simulink model "regulacion_nominal_modelo_no_lineal"  (R2021a)
settings: Solver=VariableStepAuto  StartTime=0.0  StopTime=15  RelTol=1e-3
settings Model: Creator=jmata  LastModifiedBy=jmata

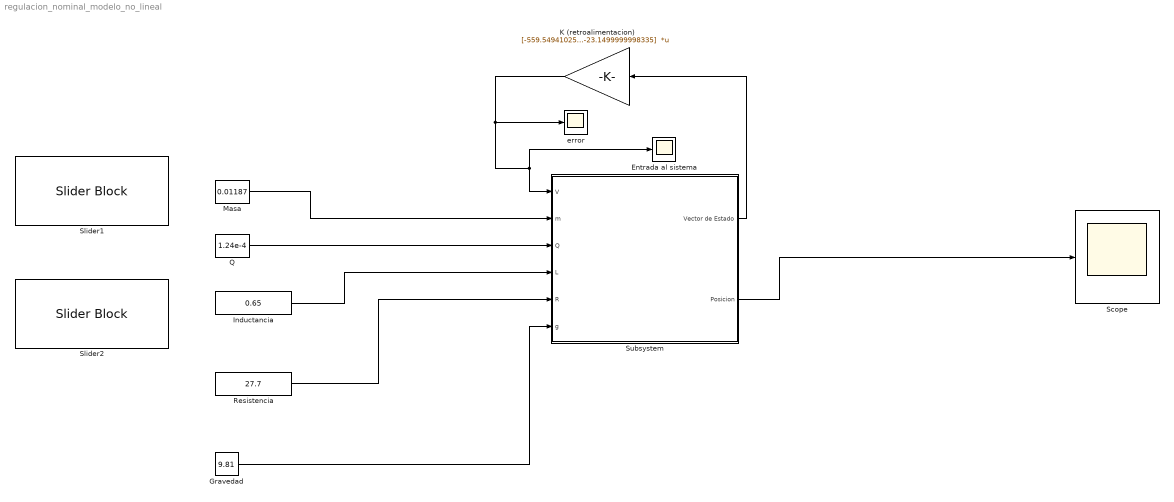
== system regulacion_nominal_modelo_no_lineal ==
  Entrada al sistema : Scope
  Gravedad : Constant  Value=9.81
  Inductancia : Constant  Value=0.65
  K (retroalimentacion) : Gain  Gain=[-559.549410259276, -81.2758440000597, -23.1499999998335]  Multiplication=Matrix(K*u)
  Masa : Constant  Value=0.01187
  Q : Constant  Value=1.24e-4
  Resistencia : Constant  Value=27.7
  Scope : Scope
  Slider1 : SliderBlock  ScaleMin=24.93  ScaleMax=30.47
  Slider2 : SliderBlock  ScaleMin=0.585  ScaleMax=0.715
  Subsystem : Subsystem
  error : Scope
  wires:
  Gravedad/1 -> Subsystem/6(g)
  Q/1 -> Subsystem/3(Q)
  Subsystem/2(Posicion) -> Scope/1
  K (retroalimentacion)/1 -> Subsystem/1(V), Entrada al sistema/1, error/1
  Subsystem/1(Vector de Estado) -> K (retroalimentacion)/1
  Resistencia/1 -> Subsystem/5(R)
  Masa/1 -> Subsystem/2(m)
  Inductancia/1 -> Subsystem/4(L)

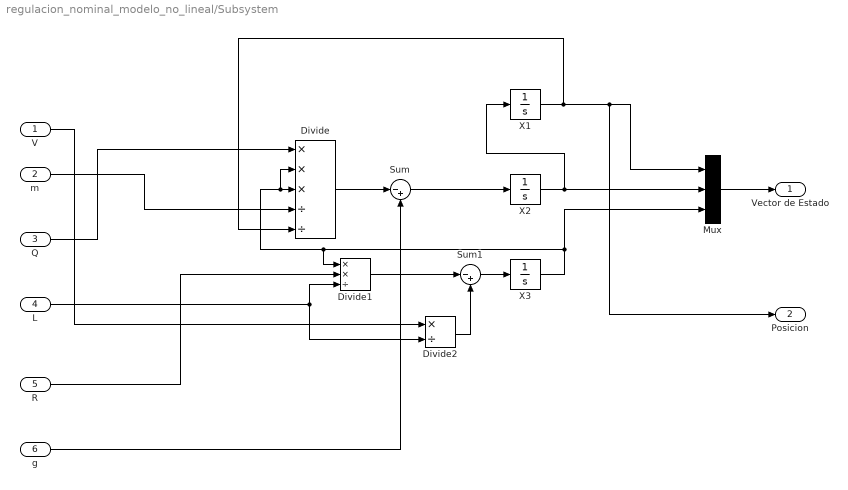
== system regulacion_nominal_modelo_no_lineal/Subsystem ==
  V : Inport
  m : Inport  Port=2
  Q : Inport  Port=3
  L : Inport  Port=4
  R : Inport  Port=5
  g : Inport  Port=6
  Divide : Product  Inputs=***//
  Divide1 : Product  Inputs=**/
  Divide2 : Product  Inputs=*/
  Mux : Mux  Inputs=3
  Sum : Sum  Inputs=|-+
  Sum1 : Sum  Inputs=|-+
  X1 : Integrator  InitialCondition=0.1
  X2 : Integrator
  X3 : Integrator
  Vector de Estado : Outport
  Posicion : Outport  Port=2
  wires:
  Divide/1 -> Sum/1
  Sum/1 -> X2/1
  L/1 -> Divide2/2, Divide1/3
  Sum1/1 -> X3/1
  X3/1 -> Mux/3, Divide1/1, Divide/2, Divide/3
  Divide2/1 -> Sum1/2
  X1/1 -> Posicion/1, Mux/1, Divide/5
  X2/1 -> Mux/2, X1/1
  g/1 -> Sum/2
  Divide1/1 -> Sum1/1
  m/1 -> Divide/4
  Q/1 -> Divide/1
  Mux/1 -> Vector de Estado/1
  R/1 -> Divide1/2
  V/1 -> Divide2/1
